simulink model "stage2_locked_interaction"  (R2026a)
settings: Solver=ode4  StopTime=stage2_stop  FixedStep=stage2_dt
undefined symbols (not defined in the file): stage2_c, stage2_k, stage2_m
settings Model: Creator=jimmy  LastModifiedBy=jimmy

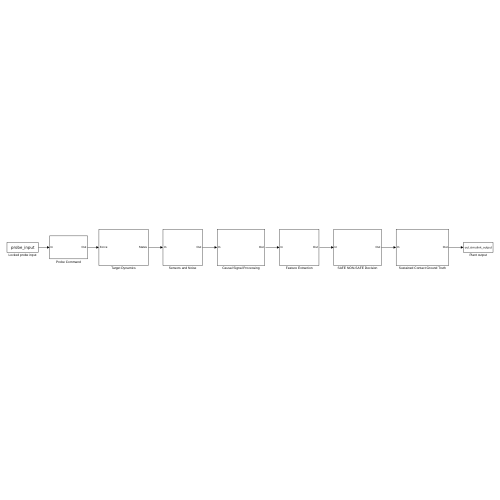
[thumbnail: Simulink's stored preview of the top-level diagram]
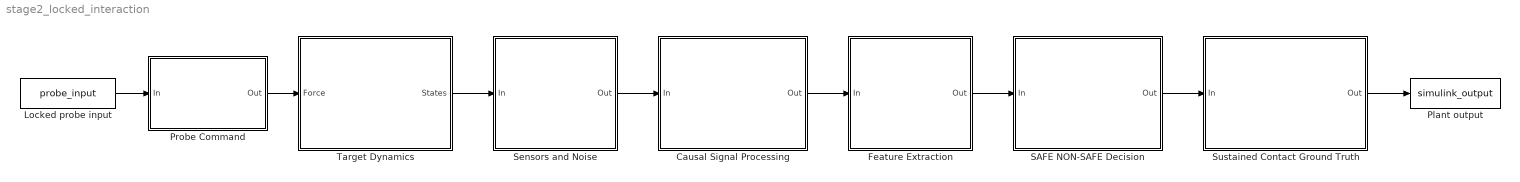
== system stage2_locked_interaction ==
  Causal Signal Processing : Subsystem
  Feature Extraction : Subsystem
  Locked probe input : FromWorkspace  VariableName=probe_input
  Plant output : ToWorkspace  SaveFormat=Timeseries  SampleTime=-1
  Probe Command : Subsystem
  SAFE NON-SAFE Decision : Subsystem
  Sensors and Noise : Subsystem
  Sustained Contact Ground Truth : Subsystem
  Target Dynamics : Subsystem
  wires:
  Locked probe input/1 -> Probe Command/1(In)
  Probe Command/1(Out) -> Target Dynamics/1(Force)
  Target Dynamics/1(States) -> Sensors and Noise/1(In)
  Sensors and Noise/1(Out) -> Causal Signal Processing/1(In)
  Causal Signal Processing/1(Out) -> Feature Extraction/1(In)
  Feature Extraction/1(Out) -> SAFE NON-SAFE Decision/1(In)
  SAFE NON-SAFE Decision/1(Out) -> Sustained Contact Ground Truth/1(In)
  Sustained Contact Ground Truth/1(Out) -> Plant output/1

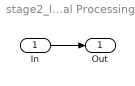
== system stage2_locked_interaction/Causal Signal Processing ==
  In : Inport
  Out : Outport
  wires:
  In/1 -> Out/1

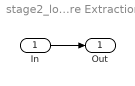
== system stage2_locked_interaction/Feature Extraction ==
  In : Inport
  Out : Outport
  wires:
  In/1 -> Out/1

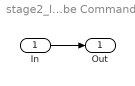
== system stage2_locked_interaction/Probe Command ==
  In : Inport
  Out : Outport
  wires:
  In/1 -> Out/1

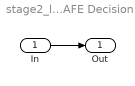
== system stage2_locked_interaction/SAFE NON-SAFE Decision ==
  In : Inport
  Out : Outport
  wires:
  In/1 -> Out/1

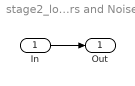
== system stage2_locked_interaction/Sensors and Noise ==
  In : Inport
  Out : Outport
  wires:
  In/1 -> Out/1

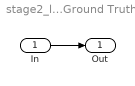
== system stage2_locked_interaction/Sustained Contact Ground Truth ==
  In : Inport
  Out : Outport
  wires:
  In/1 -> Out/1

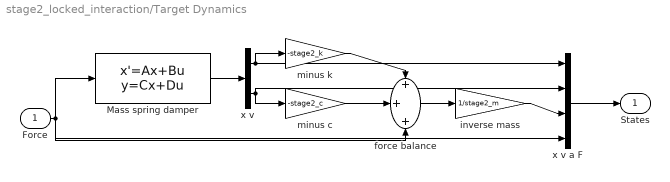
== system stage2_locked_interaction/Target Dynamics ==
  Force : Inport
  Mass spring damper : StateSpace  A=[0 1;-stage2_k/stage2_m -stage2_c/stage2_m]  B=[0;1/stage2_m]  C=eye(2)  D=[0;0]  InitialCondition=[0;0]
  force balance : Sum  Inputs=+++
  inverse mass : Gain  Gain=1/stage2_m
  minus c : Gain  Gain=-stage2_c
  minus k : Gain  Gain=-stage2_k
  x v : Demux  Outputs=2
  x v a F : Mux
  States : Outport
  wires:
  Force/1 -> Mass spring damper/1, force balance/3, x v a F/4
  Mass spring damper/1 -> x v/1
  x v/1 -> minus k/1, x v a F/1
  x v/2 -> minus c/1, x v a F/2
  minus k/1 -> force balance/1
  minus c/1 -> force balance/2
  force balance/1 -> inverse mass/1
  inverse mass/1 -> x v a F/3
  x v a F/1 -> States/1
